simulink model "OMSv1_4"  (Simulink 7.0)
settings: Solver=ode4  SolverMode=SingleTasking  StartTime=0.0  StopTime=4  FixedStep=0.001  MaxStep=0.001  RelTol=1e-3  AbsTol=1e-3
PreLoadFcn:
  | setmdlp
values from neighbouring files (symbols this model uses):
  mdlparamlist = loadin.old    [setmdlp.m]
undefined symbols (not defined in the file or in its folder): alexlaw, bs_onoff, bs_scale, bsfsacrit, bsfsvcrit, cnsgain, current, fs_onoff, fs_scale, fsdelaycalc, ltdrk, phasicgain, pmcgain, pmctau2, pmctau3, saccsw, sigbuilder_block, spgain, tonicgain, tvrD, tvrN
(part 9 of 10)

== system OMSv1_4/OMS v1.4  12/31/07/IM CN-LMLN/Sampled Target Reconstruction/prolong/trailing edge detect/Sign ==
  in_1 : Inport  OutDataType=sfix(16)  OutScaling=2^0
  Constant : Constant  Value=0  OutDataType=sfix(16)  OutScaling=2^0
  Relational Operator : RelationalOperator  Operator=>  InputSameDT=on
  Relational Operator1 : RelationalOperator  Operator=<  InputSameDT=on
  Sum : Sum  Inputs=+-  OutDataType=sfix(16)  OutScaling=2^0  SaturateOnIntegerOverflow=on  InputSameDT=on
  out_1 : Outport  OutDataType=sfix(16)  OutScaling=2^0  InitialOutput=0
  wires:
  in_1/1 -> Relational Operator/1, Relational Operator1/1
  Constant/1 -> Relational Operator1/2, Relational Operator/2
  Relational Operator1/1 -> Sum/2
  Relational Operator/1 -> Sum/1
  Sum/1 -> out_1/1

== system OMSv1_4/OMS v1.4  12/31/07/IM CN-LMLN/Sampled Target Reconstruction/prolong1/SampHold?2/Sign ==
  in_1 : Inport  OutDataType=sfix(16)  OutScaling=2^0
  Constant : Constant  Value=0  OutDataType=sfix(16)  OutScaling=2^0
  Relational Operator : RelationalOperator  Operator=>  InputSameDT=on
  Relational Operator1 : RelationalOperator  Operator=<  InputSameDT=on
  Sum : Sum  Inputs=+-  OutDataType=sfix(16)  OutScaling=2^0  SaturateOnIntegerOverflow=on  InputSameDT=on
  out_1 : Outport  OutDataType=sfix(16)  OutScaling=2^0  InitialOutput=0
  wires:
  Sum/1 -> out_1/1
  Relational Operator/1 -> Sum/1
  Relational Operator1/1 -> Sum/2
  Constant/1 -> Relational Operator/2, Relational Operator1/2
  in_1/1 -> Relational Operator1/1, Relational Operator/1

== system OMSv1_4/OMS v1.4  12/31/07/IM CN-LMLN/Sampled Target Reconstruction/prolong1/leading edge detect/Sign ==
  in_1 : Inport  OutDataType=sfix(16)  OutScaling=2^0
  Constant : Constant  Value=0  OutDataType=sfix(16)  OutScaling=2^0
  Relational Operator : RelationalOperator  Operator=>  InputSameDT=on
  Relational Operator1 : RelationalOperator  Operator=<  InputSameDT=on
  Sum : Sum  Inputs=+-  OutDataType=sfix(16)  OutScaling=2^0  SaturateOnIntegerOverflow=on  InputSameDT=on
  out_1 : Outport  OutDataType=sfix(16)  OutScaling=2^0  InitialOutput=0
  wires:
  in_1/1 -> Relational Operator/1, Relational Operator1/1
  Constant/1 -> Relational Operator1/2, Relational Operator/2
  Relational Operator1/1 -> Sum/2
  Relational Operator/1 -> Sum/1
  Sum/1 -> out_1/1

== system OMSv1_4/OMS v1.4  12/31/07/IM CN-LMLN/Sampled Target Reconstruction/prolong1/trailing edge detect/Sign ==
  in_1 : Inport  OutDataType=sfix(16)  OutScaling=2^0
  Constant : Constant  Value=0  OutDataType=sfix(16)  OutScaling=2^0
  Relational Operator : RelationalOperator  Operator=>  InputSameDT=on
  Relational Operator1 : RelationalOperator  Operator=<  InputSameDT=on
  Sum : Sum  Inputs=+-  OutDataType=sfix(16)  OutScaling=2^0  SaturateOnIntegerOverflow=on  InputSameDT=on
  out_1 : Outport  OutDataType=sfix(16)  OutScaling=2^0  InitialOutput=0
  wires:
  Sum/1 -> out_1/1
  Relational Operator/1 -> Sum/1
  Relational Operator1/1 -> Sum/2
  Constant/1 -> Relational Operator/2, Relational Operator1/2
  in_1/1 -> Relational Operator1/1, Relational Operator/1

== system OMSv1_4/OMS v1.4  12/31/07/IM CN-LMLN/Sampled Target Reconstruction/prolong2/SampHold?2/Sign ==
  in_1 : Inport  OutDataType=sfix(16)  OutScaling=2^0
  Constant : Constant  Value=0  OutDataType=sfix(16)  OutScaling=2^0
  Relational Operator : RelationalOperator  Operator=>  InputSameDT=on
  Relational Operator1 : RelationalOperator  Operator=<  InputSameDT=on
  Sum : Sum  Inputs=+-  OutDataType=sfix(16)  OutScaling=2^0  SaturateOnIntegerOverflow=on  InputSameDT=on
  out_1 : Outport  OutDataType=sfix(16)  OutScaling=2^0  InitialOutput=0
  wires:
  in_1/1 -> Relational Operator/1, Relational Operator1/1
  Constant/1 -> Relational Operator1/2, Relational Operator/2
  Relational Operator1/1 -> Sum/2
  Relational Operator/1 -> Sum/1
  Sum/1 -> out_1/1

== system OMSv1_4/OMS v1.4  12/31/07/IM CN-LMLN/Sampled Target Reconstruction/prolong2/leading edge detect/Sign ==
  in_1 : Inport  OutDataType=sfix(16)  OutScaling=2^0
  Constant : Constant  Value=0  OutDataType=sfix(16)  OutScaling=2^0
  Relational Operator : RelationalOperator  Operator=>  InputSameDT=on
  Relational Operator1 : RelationalOperator  Operator=<  InputSameDT=on
  Sum : Sum  Inputs=+-  OutDataType=sfix(16)  OutScaling=2^0  SaturateOnIntegerOverflow=on  InputSameDT=on
  out_1 : Outport  OutDataType=sfix(16)  OutScaling=2^0  InitialOutput=0
  wires:
  Sum/1 -> out_1/1
  Relational Operator/1 -> Sum/1
  Relational Operator1/1 -> Sum/2
  Constant/1 -> Relational Operator/2, Relational Operator1/2
  in_1/1 -> Relational Operator1/1, Relational Operator/1

== system OMSv1_4/OMS v1.4  12/31/07/IM CN-LMLN/Sampled Target Reconstruction/prolong2/trailing edge detect/Sign ==
  in_1 : Inport  OutDataType=sfix(16)  OutScaling=2^0
  Constant : Constant  Value=0  OutDataType=sfix(16)  OutScaling=2^0
  Relational Operator : RelationalOperator  Operator=>  InputSameDT=on
  Relational Operator1 : RelationalOperator  Operator=<  InputSameDT=on
  Sum : Sum  Inputs=+-  OutDataType=sfix(16)  OutScaling=2^0  SaturateOnIntegerOverflow=on  InputSameDT=on
  out_1 : Outport  OutDataType=sfix(16)  OutScaling=2^0  InitialOutput=0
  wires:
  in_1/1 -> Relational Operator/1, Relational Operator1/1
  Constant/1 -> Relational Operator1/2, Relational Operator/2
  Relational Operator1/1 -> Sum/2
  Relational Operator/1 -> Sum/1
  Sum/1 -> out_1/1

== system OMSv1_4/OMS v1.4  12/31/07/PG w rNI2/PW funct/Input Switch/lead/trail edge det/Sign ==
  in_1 : Inport  OutDataType=sfix(16)  OutScaling=2^0
  Constant : Constant  Value=0  OutDataType=sfix(16)  OutScaling=2^0
  Relational Operator : RelationalOperator  Operator=>  InputSameDT=on
  Relational Operator1 : RelationalOperator  Operator=<  InputSameDT=on
  Sum : Sum  Inputs=+-  OutDataType=sfix(16)  OutScaling=2^0  SaturateOnIntegerOverflow=on  InputSameDT=on
  out_1 : Outport  OutDataType=sfix(16)  OutScaling=2^0  InitialOutput=0
  wires:
  in_1/1 -> Relational Operator/1, Relational Operator1/1
  Constant/1 -> Relational Operator1/2, Relational Operator/2
  Relational Operator1/1 -> Sum/2
  Relational Operator/1 -> Sum/1
  Sum/1 -> out_1/1

== system OMSv1_4/OMS v1.4  12/31/07/PG w rNI2/RefLatch (Default = 50ms)/trailing edge/trailing edge det/Sign ==
  in_1 : Inport  OutDataType=sfix(16)  OutScaling=2^0
  Constant : Constant  Value=0  OutDataType=sfix(16)  OutScaling=2^0
  Relational Operator : RelationalOperator  Operator=>  InputSameDT=on
  Relational Operator1 : RelationalOperator  Operator=<  InputSameDT=on
  Sum : Sum  Inputs=+-  OutDataType=sfix(16)  OutScaling=2^0  SaturateOnIntegerOverflow=on  InputSameDT=on
  out_1 : Outport  OutDataType=sfix(16)  OutScaling=2^0  InitialOutput=0
  wires:
  in_1/1 -> Relational Operator/1, Relational Operator1/1
  Constant/1 -> Relational Operator1/2, Relational Operator/2
  Relational Operator1/1 -> Sum/2
  Relational Operator/1 -> Sum/1
  Sum/1 -> out_1/1

== system OMSv1_4/OMS v1.4  12/31/07/PG w rNI2/RefLatch (Default = 50ms)/trailing edge/trailing edge det1/Sign ==
  in_1 : Inport  OutDataType=sfix(16)  OutScaling=2^0
  Constant : Constant  Value=0  OutDataType=sfix(16)  OutScaling=2^0
  Relational Operator : RelationalOperator  Operator=>  InputSameDT=on
  Relational Operator1 : RelationalOperator  Operator=<  InputSameDT=on
  Sum : Sum  Inputs=+-  OutDataType=sfix(16)  OutScaling=2^0  SaturateOnIntegerOverflow=on  InputSameDT=on
  out_1 : Outport  OutDataType=sfix(16)  OutScaling=2^0  InitialOutput=0
  wires:
  Sum/1 -> out_1/1
  Relational Operator/1 -> Sum/1
  Relational Operator1/1 -> Sum/2
  Constant/1 -> Relational Operator1/2, Relational Operator/2
  in_1/1 -> Relational Operator/1, Relational Operator1/1

== system OMSv1_4/OMS v1.4  12/31/07/IM CN-LMLN/BS/FS Logic/BS Enable1/BS Timing/event timer2/Latch1 ==
  in_1 : Inport  OutDataType=sfix(16)  OutScaling=2^0
  in_2 : Inport  Port=2  OutDataType=sfix(16)  OutScaling=2^0
  Demux : Demux  Outputs=2
  Logic : CombinatorialLogic  TruthTable=[0 1;0 1;1 0;0 1;1 0;0 1;1 0;1 0]
  Memory : Memory  Orientation=left  X0=ini
  Mux : Mux  Inputs=3
  out_1 : Outport  OutDataType=sfix(16)  OutScaling=2^0  InitialOutput=0
  out_2 : Outport  Port=2  OutDataType=sfix(16)  OutScaling=2^0  InitialOutput=0
  wires:
  in_2/1 -> Mux/3
  in_1/1 -> Mux/2
  Memory/1 -> Mux/1
  Demux/1 -> Memory/1, out_1/1
  Mux/1 -> Logic/1
  Logic/1 -> Demux/1
  Demux/2 -> out_2/1

== system OMSv1_4/OMS v1.4  12/31/07/IM CN-LMLN/BS/FS Logic/BS Enable1/BS Timing/event timer2/SampHold?1 ==
  note: When "S/H?" is LOW, then "Input" is switched directly to the
      | output ("sample").  When "S/H?" is HIGH, the current output is
      | maintained ("hold").
  Input : Inport  OutDataType=sfix(16)  OutScaling=2^0
  S/H? : Inport  Port=2  OutDataType=sfix(16)  OutScaling=2^0
  Memory : Memory  Orientation=left
  Sign : Subsystem
      mask Type: Sign
      mask Description: y = sign(x)
      mask Help: Sign Function:\n\t\t\ty = 1 if x > 0\n\t\t\ty = 0 if x = 0\n\t\t\ty = -1 if x < 0
      mask Display: plot(-50,-50,50,50,[-50,50],[0,0],[0,0],[-50,50],[-40,0],[-30,-30],[0,40],[30,30])
  Switch2 : Switch  Threshold=0.5  SaturateOnIntegerOverflow=on  InputSameDT=on
  output : Outport  OutDataType=sfix(16)  OutScaling=2^0  InitialOutput=0
  wires:
  Switch2/1 -> Memory/1, output/1
  Sign/1(out_1) -> Switch2/2
  S/H?/1 -> Sign/1(in_1)
  Memory/1 -> Switch2/1
  Input/1 -> Switch2/3

== system OMSv1_4/OMS v1.4  12/31/07/IM CN-LMLN/BS/FS Logic/BS Enable1/BS Timing/event timer2/leading edge detect ==
  note: It is also possible to remove the SIGNUM function
      | and the '==', and replace them with a simple
      | switch with a threshold of (say) 150 or so.
  note: leading edge detection
  in_1 : Inport  OutDataType=sfix(16)  OutScaling=2^0
  Abs : Abs  SaturateOnIntegerOverflow=on
  Derivative : Derivative
  Relational Operator : RelationalOperator  Operator===  InputSameDT=on
  Sign : Subsystem
      mask Type: Sign
      mask Description: y = sign(x)
      mask Help: Sign Function:\n\t\t\ty = 1 if x > 0\n\t\t\ty = 0 if x = 0\n\t\t\ty = -1 if x < 0
      mask Display: plot(-50,-50,50,50,[-50,50],[0,0],[0,0],[-50,50],[-40,0],[-30,-30],[0,40],[30,30])
  Threshold 1 : Constant  OutDataType=sfix(16)  OutScaling=2^0
  out_1 : Outport  OutDataType=sfix(16)  OutScaling=2^0  InitialOutput=0
  wires:
  Abs/1 -> Derivative/1
  Derivative/1 -> Sign/1(in_1)
  Sign/1(out_1) -> Relational Operator/1
  Threshold 1/1 -> Relational Operator/2
  Relational Operator/1 -> out_1/1
  in_1/1 -> Abs/1

== system OMSv1_4/OMS v1.4  12/31/07/IM CN-LMLN/BS/FS Logic/BS Enable1/BS Timing/event timer2/trailing edge detect ==
  note: trailing edge detection
  note: It is also possible to remove the SIGNUM function
      | and the '==', and replace them with a simple
      | switch with a threshold of (say) 150 or so.
  in_1 : Inport  OutDataType=sfix(16)  OutScaling=2^0
  Abs : Abs  SaturateOnIntegerOverflow=on
  Derivative : Derivative
  Relational Operator : RelationalOperator  Operator===  InputSameDT=on
  Sign : Subsystem
      mask Type: Sign
      mask Description: y = sign(x)
      mask Help: Sign Function:\n\t\t\ty = 1 if x > 0\n\t\t\ty = 0 if x = 0\n\t\t\ty = -1 if x < 0
      mask Display: plot(-50,-50,50,50,[-50,50],[0,0],[0,0],[-50,50],[-40,0],[-30,-30],[0,40],[30,30])
  Threshold 1 : Constant  Value=-1  OutDataType=sfix(16)  OutScaling=2^0
  out_1 : Outport  OutDataType=sfix(16)  OutScaling=2^0  InitialOutput=0
  wires:
  in_1/1 -> Abs/1
  Relational Operator/1 -> out_1/1
  Threshold 1/1 -> Relational Operator/2
  Sign/1(out_1) -> Relational Operator/1
  Derivative/1 -> Sign/1(in_1)
  Abs/1 -> Derivative/1

== system OMSv1_4/OMS v1.4  12/31/07/IM CN-LMLN/BS/FS Logic/BS Enable1/BS Timing/leading edge detect/Sign ==
  in_1 : Inport  OutDataType=sfix(16)  OutScaling=2^0
  Constant : Constant  Value=0  OutDataType=sfix(16)  OutScaling=2^0
  Relational Operator : RelationalOperator  Operator=>  InputSameDT=on
  Relational Operator1 : RelationalOperator  Operator=<  InputSameDT=on
  Sum : Sum  Inputs=+-  OutDataType=sfix(16)  OutScaling=2^0  SaturateOnIntegerOverflow=on  InputSameDT=on
  out_1 : Outport  OutDataType=sfix(16)  OutScaling=2^0  InitialOutput=0
  wires:
  Sum/1 -> out_1/1
  Relational Operator/1 -> Sum/1
  Relational Operator1/1 -> Sum/2
  Constant/1 -> Relational Operator/2, Relational Operator1/2
  in_1/1 -> Relational Operator1/1, Relational Operator/1

== system OMSv1_4/OMS v1.4  12/31/07/IM CN-LMLN/BS/FS Logic/FS Enable/FS Timing/event timer2/Latch1 ==
  in_1 : Inport  OutDataType=sfix(16)  OutScaling=2^0
  in_2 : Inport  Port=2  OutDataType=sfix(16)  OutScaling=2^0
  Demux : Demux  Outputs=2
  Logic : CombinatorialLogic  TruthTable=[0 1;0 1;1 0;0 1;1 0;0 1;1 0;1 0]
  Memory : Memory  Orientation=left  X0=ini
  Mux : Mux  Inputs=3
  out_1 : Outport  OutDataType=sfix(16)  OutScaling=2^0  InitialOutput=0
  out_2 : Outport  Port=2  OutDataType=sfix(16)  OutScaling=2^0  InitialOutput=0
  wires:
  Demux/2 -> out_2/1
  Logic/1 -> Demux/1
  Mux/1 -> Logic/1
  Demux/1 -> out_1/1, Memory/1
  Memory/1 -> Mux/1
  in_1/1 -> Mux/2
  in_2/1 -> Mux/3

== system OMSv1_4/OMS v1.4  12/31/07/IM CN-LMLN/BS/FS Logic/FS Enable/FS Timing/event timer2/SampHold?1 ==
  note: When "S/H?" is LOW, then "Input" is switched directly to the
      | output ("sample").  When "S/H?" is HIGH, the current output is
      | maintained ("hold").
  Input : Inport  OutDataType=sfix(16)  OutScaling=2^0
  S/H? : Inport  Port=2  OutDataType=sfix(16)  OutScaling=2^0
  Memory : Memory  Orientation=left
  Sign : Subsystem
      mask Type: Sign
      mask Description: y = sign(x)
      mask Help: Sign Function:\n\t\t\ty = 1 if x > 0\n\t\t\ty = 0 if x = 0\n\t\t\ty = -1 if x < 0
      mask Display: plot(-50,-50,50,50,[-50,50],[0,0],[0,0],[-50,50],[-40,0],[-30,-30],[0,40],[30,30])
  Switch2 : Switch  Threshold=0.5  SaturateOnIntegerOverflow=on  InputSameDT=on
  output : Outport  OutDataType=sfix(16)  OutScaling=2^0  InitialOutput=0
  wires:
  Input/1 -> Switch2/3
  Memory/1 -> Switch2/1
  S/H?/1 -> Sign/1(in_1)
  Sign/1(out_1) -> Switch2/2
  Switch2/1 -> output/1, Memory/1

== system OMSv1_4/OMS v1.4  12/31/07/IM CN-LMLN/BS/FS Logic/FS Enable/FS Timing/event timer2/leading edge detect ==
  note: leading edge detection
  note: It is also possible to remove the SIGNUM function
      | and the '==', and replace them with a simple
      | switch with a threshold of (say) 150 or so.
  in_1 : Inport  OutDataType=sfix(16)  OutScaling=2^0
  Abs : Abs  SaturateOnIntegerOverflow=on
  Derivative : Derivative
  Relational Operator : RelationalOperator  Operator===  InputSameDT=on
  Sign : Subsystem
      mask Type: Sign
      mask Description: y = sign(x)
      mask Help: Sign Function:\n\t\t\ty = 1 if x > 0\n\t\t\ty = 0 if x = 0\n\t\t\ty = -1 if x < 0
      mask Display: plot(-50,-50,50,50,[-50,50],[0,0],[0,0],[-50,50],[-40,0],[-30,-30],[0,40],[30,30])
  Threshold 1 : Constant  OutDataType=sfix(16)  OutScaling=2^0
  out_1 : Outport  OutDataType=sfix(16)  OutScaling=2^0  InitialOutput=0
  wires:
  in_1/1 -> Abs/1
  Relational Operator/1 -> out_1/1
  Threshold 1/1 -> Relational Operator/2
  Sign/1(out_1) -> Relational Operator/1
  Derivative/1 -> Sign/1(in_1)
  Abs/1 -> Derivative/1

== system OMSv1_4/OMS v1.4  12/31/07/IM CN-LMLN/BS/FS Logic/FS Enable/FS Timing/event timer2/trailing edge detect ==
  note: It is also possible to remove the SIGNUM function
      | and the '==', and replace them with a simple
      | switch with a threshold of (say) 150 or so.
  note: trailing edge detection
  in_1 : Inport  OutDataType=sfix(16)  OutScaling=2^0
  Abs : Abs  SaturateOnIntegerOverflow=on
  Derivative : Derivative
  Relational Operator : RelationalOperator  Operator===  InputSameDT=on
  Sign : Subsystem
      mask Type: Sign
      mask Description: y = sign(x)
      mask Help: Sign Function:\n\t\t\ty = 1 if x > 0\n\t\t\ty = 0 if x = 0\n\t\t\ty = -1 if x < 0
      mask Display: plot(-50,-50,50,50,[-50,50],[0,0],[0,0],[-50,50],[-40,0],[-30,-30],[0,40],[30,30])
  Threshold 1 : Constant  Value=-1  OutDataType=sfix(16)  OutScaling=2^0
  out_1 : Outport  OutDataType=sfix(16)  OutScaling=2^0  InitialOutput=0
  wires:
  Abs/1 -> Derivative/1
  Derivative/1 -> Sign/1(in_1)
  Sign/1(out_1) -> Relational Operator/1
  Threshold 1/1 -> Relational Operator/2
  Relational Operator/1 -> out_1/1
  in_1/1 -> Abs/1

== system OMSv1_4/OMS v1.4  12/31/07/IM CN-LMLN/BS/FS Logic/FS Enable/FS Timing/leading edge detect/Sign ==
  in_1 : Inport  OutDataType=sfix(16)  OutScaling=2^0
  Constant : Constant  Value=0  OutDataType=sfix(16)  OutScaling=2^0
  Relational Operator : RelationalOperator  Operator=>  InputSameDT=on
  Relational Operator1 : RelationalOperator  Operator=<  InputSameDT=on
  Sum : Sum  Inputs=+-  OutDataType=sfix(16)  OutScaling=2^0  SaturateOnIntegerOverflow=on  InputSameDT=on
  out_1 : Outport  OutDataType=sfix(16)  OutScaling=2^0  InitialOutput=0
  wires:
  in_1/1 -> Relational Operator/1, Relational Operator1/1
  Constant/1 -> Relational Operator1/2, Relational Operator/2
  Relational Operator1/1 -> Sum/2
  Relational Operator/1 -> Sum/1
  Sum/1 -> out_1/1

== system OMSv1_4/OMS v1.4  12/31/07/IM CN-LMLN/BS/FS Logic/FS Enable/prolong/SampHold?2/Sign ==
  in_1 : Inport  OutDataType=sfix(16)  OutScaling=2^0
  Constant : Constant  Value=0  OutDataType=sfix(16)  OutScaling=2^0
  Relational Operator : RelationalOperator  Operator=>  InputSameDT=on
  Relational Operator1 : RelationalOperator  Operator=<  InputSameDT=on
  Sum : Sum  Inputs=+-  OutDataType=sfix(16)  OutScaling=2^0  SaturateOnIntegerOverflow=on  InputSameDT=on
  out_1 : Outport  OutDataType=sfix(16)  OutScaling=2^0  InitialOutput=0
  wires:
  in_1/1 -> Relational Operator/1, Relational Operator1/1
  Constant/1 -> Relational Operator1/2, Relational Operator/2
  Relational Operator1/1 -> Sum/2
  Relational Operator/1 -> Sum/1
  Sum/1 -> out_1/1

== system OMSv1_4/OMS v1.4  12/31/07/IM CN-LMLN/BS/FS Logic/FS Enable/prolong/leading edge detect/Sign ==
  in_1 : Inport  OutDataType=sfix(16)  OutScaling=2^0
  Constant : Constant  Value=0  OutDataType=sfix(16)  OutScaling=2^0
  Relational Operator : RelationalOperator  Operator=>  InputSameDT=on
  Relational Operator1 : RelationalOperator  Operator=<  InputSameDT=on
  Sum : Sum  Inputs=+-  OutDataType=sfix(16)  OutScaling=2^0  SaturateOnIntegerOverflow=on  InputSameDT=on
  out_1 : Outport  OutDataType=sfix(16)  OutScaling=2^0  InitialOutput=0
  wires:
  Sum/1 -> out_1/1
  Relational Operator/1 -> Sum/1
  Relational Operator1/1 -> Sum/2
  Constant/1 -> Relational Operator/2, Relational Operator1/2
  in_1/1 -> Relational Operator1/1, Relational Operator/1

== system OMSv1_4/OMS v1.4  12/31/07/IM CN-LMLN/BS/FS Logic/FS Enable/prolong/trailing edge detect/Sign ==
  in_1 : Inport  OutDataType=sfix(16)  OutScaling=2^0
  Constant : Constant  Value=0  OutDataType=sfix(16)  OutScaling=2^0
  Relational Operator : RelationalOperator  Operator=>  InputSameDT=on
  Relational Operator1 : RelationalOperator  Operator=<  InputSameDT=on
  Sum : Sum  Inputs=+-  OutDataType=sfix(16)  OutScaling=2^0  SaturateOnIntegerOverflow=on  InputSameDT=on
  out_1 : Outport  OutDataType=sfix(16)  OutScaling=2^0  InitialOutput=0
  wires:
  in_1/1 -> Relational Operator/1, Relational Operator1/1
  Constant/1 -> Relational Operator1/2, Relational Operator/2
  Relational Operator1/1 -> Sum/2
  Relational Operator/1 -> Sum/1
  Sum/1 -> out_1/1

== system OMSv1_4/OMS v1.4  12/31/07/IM CN-LMLN/BS/FS Logic/TCHNG Override/event timer2/SampHold?1/Sign ==
  in_1 : Inport  OutDataType=sfix(16)  OutScaling=2^0
  Constant : Constant  Value=0  OutDataType=sfix(16)  OutScaling=2^0
  Relational Operator : RelationalOperator  Operator=>  InputSameDT=on
  Relational Operator1 : RelationalOperator  Operator=<  InputSameDT=on
  Sum : Sum  Inputs=+-  OutDataType=sfix(16)  OutScaling=2^0  SaturateOnIntegerOverflow=on  InputSameDT=on
  out_1 : Outport  OutDataType=sfix(16)  OutScaling=2^0  InitialOutput=0
  wires:
  in_1/1 -> Relational Operator1/1, Relational Operator/1
  Constant/1 -> Relational Operator/2, Relational Operator1/2
  Relational Operator1/1 -> Sum/2
  Relational Operator/1 -> Sum/1
  Sum/1 -> out_1/1

== system OMSv1_4/OMS v1.4  12/31/07/IM CN-LMLN/BS/FS Logic/TCHNG Override/event timer2/leading edge detect/Sign ==
  in_1 : Inport  OutDataType=sfix(16)  OutScaling=2^0
  Constant : Constant  Value=0  OutDataType=sfix(16)  OutScaling=2^0
  Relational Operator : RelationalOperator  Operator=>  InputSameDT=on
  Relational Operator1 : RelationalOperator  Operator=<  InputSameDT=on
  Sum : Sum  Inputs=+-  OutDataType=sfix(16)  OutScaling=2^0  SaturateOnIntegerOverflow=on  InputSameDT=on
  out_1 : Outport  OutDataType=sfix(16)  OutScaling=2^0  InitialOutput=0
  wires:
  in_1/1 -> Relational Operator1/1, Relational Operator/1
  Constant/1 -> Relational Operator/2, Relational Operator1/2
  Relational Operator1/1 -> Sum/2
  Relational Operator/1 -> Sum/1
  Sum/1 -> out_1/1

== system OMSv1_4/OMS v1.4  12/31/07/IM CN-LMLN/BS/FS Logic/TCHNG Override/event timer2/trailing edge detect/Sign ==
  in_1 : Inport  OutDataType=sfix(16)  OutScaling=2^0
  Constant : Constant  Value=0  OutDataType=sfix(16)  OutScaling=2^0
  Relational Operator : RelationalOperator  Operator=>  InputSameDT=on
  Relational Operator1 : RelationalOperator  Operator=<  InputSameDT=on
  Sum : Sum  Inputs=+-  OutDataType=sfix(16)  OutScaling=2^0  SaturateOnIntegerOverflow=on  InputSameDT=on
  out_1 : Outport  OutDataType=sfix(16)  OutScaling=2^0  InitialOutput=0
  wires:
  Sum/1 -> out_1/1
  Relational Operator/1 -> Sum/1
  Relational Operator1/1 -> Sum/2
  Constant/1 -> Relational Operator/2, Relational Operator1/2
  in_1/1 -> Relational Operator1/1, Relational Operator/1

== system OMSv1_4/OMS v1.4  12/31/07/IM CN-LMLN/Saccade Enable/Enable Control/2 ms/SampHold?2/Sign ==
  in_1 : Inport  OutDataType=sfix(16)  OutScaling=2^0
  Constant : Constant  Value=0  OutDataType=sfix(16)  OutScaling=2^0
  Relational Operator : RelationalOperator  Operator=>  InputSameDT=on
  Relational Operator1 : RelationalOperator  Operator=<  InputSameDT=on
  Sum : Sum  Inputs=+-  OutDataType=sfix(16)  OutScaling=2^0  SaturateOnIntegerOverflow=on  InputSameDT=on
  out_1 : Outport  OutDataType=sfix(16)  OutScaling=2^0  InitialOutput=0
  wires:
  Sum/1 -> out_1/1
  Relational Operator/1 -> Sum/1
  Relational Operator1/1 -> Sum/2
  Constant/1 -> Relational Operator/2, Relational Operator1/2
  in_1/1 -> Relational Operator1/1, Relational Operator/1

== system OMSv1_4/OMS v1.4  12/31/07/IM CN-LMLN/Saccade Enable/Enable Control/2 ms/leading edge detect/Sign ==
  in_1 : Inport  OutDataType=sfix(16)  OutScaling=2^0
  Constant : Constant  Value=0  OutDataType=sfix(16)  OutScaling=2^0
  Relational Operator : RelationalOperator  Operator=>  InputSameDT=on
  Relational Operator1 : RelationalOperator  Operator=<  InputSameDT=on
  Sum : Sum  Inputs=+-  OutDataType=sfix(16)  OutScaling=2^0  SaturateOnIntegerOverflow=on  InputSameDT=on
  out_1 : Outport  OutDataType=sfix(16)  OutScaling=2^0  InitialOutput=0
  wires:
  in_1/1 -> Relational Operator/1, Relational Operator1/1
  Constant/1 -> Relational Operator1/2, Relational Operator/2
  Relational Operator1/1 -> Sum/2
  Relational Operator/1 -> Sum/1
  Sum/1 -> out_1/1

== system OMSv1_4/OMS v1.4  12/31/07/IM CN-LMLN/Saccade Enable/Enable Control/2 ms/trailing edge detect/Sign ==
  in_1 : Inport  OutDataType=sfix(16)  OutScaling=2^0
  Constant : Constant  Value=0  OutDataType=sfix(16)  OutScaling=2^0
  Relational Operator : RelationalOperator  Operator=>  InputSameDT=on
  Relational Operator1 : RelationalOperator  Operator=<  InputSameDT=on
  Sum : Sum  Inputs=+-  OutDataType=sfix(16)  OutScaling=2^0  SaturateOnIntegerOverflow=on  InputSameDT=on
  out_1 : Outport  OutDataType=sfix(16)  OutScaling=2^0  InitialOutput=0
  wires:
  Sum/1 -> out_1/1
  Relational Operator/1 -> Sum/1
  Relational Operator1/1 -> Sum/2
  Constant/1 -> Relational Operator/2, Relational Operator1/2
  in_1/1 -> Relational Operator1/1, Relational Operator/1

== system OMSv1_4/OMS v1.4  12/31/07/IM CN-LMLN/Saccade Enable/Enable Control/50 ms/SampHold?2/Sign ==
  in_1 : Inport  OutDataType=sfix(16)  OutScaling=2^0
  Constant : Constant  Value=0  OutDataType=sfix(16)  OutScaling=2^0
  Relational Operator : RelationalOperator  Operator=>  InputSameDT=on
  Relational Operator1 : RelationalOperator  Operator=<  InputSameDT=on
  Sum : Sum  Inputs=+-  OutDataType=sfix(16)  OutScaling=2^0  SaturateOnIntegerOverflow=on  InputSameDT=on
  out_1 : Outport  OutDataType=sfix(16)  OutScaling=2^0  InitialOutput=0
  wires:
  in_1/1 -> Relational Operator/1, Relational Operator1/1
  Constant/1 -> Relational Operator1/2, Relational Operator/2
  Relational Operator1/1 -> Sum/2
  Relational Operator/1 -> Sum/1
  Sum/1 -> out_1/1

== system OMSv1_4/OMS v1.4  12/31/07/IM CN-LMLN/Saccade Enable/Enable Control/50 ms/leading edge detect/Sign ==
  in_1 : Inport  OutDataType=sfix(16)  OutScaling=2^0
  Constant : Constant  Value=0  OutDataType=sfix(16)  OutScaling=2^0
  Relational Operator : RelationalOperator  Operator=>  InputSameDT=on
  Relational Operator1 : RelationalOperator  Operator=<  InputSameDT=on
  Sum : Sum  Inputs=+-  OutDataType=sfix(16)  OutScaling=2^0  SaturateOnIntegerOverflow=on  InputSameDT=on
  out_1 : Outport  OutDataType=sfix(16)  OutScaling=2^0  InitialOutput=0
  wires:
  Sum/1 -> out_1/1
  Relational Operator/1 -> Sum/1
  Relational Operator1/1 -> Sum/2
  Constant/1 -> Relational Operator/2, Relational Operator1/2
  in_1/1 -> Relational Operator1/1, Relational Operator/1

== system OMSv1_4/OMS v1.4  12/31/07/IM CN-LMLN/Saccade Enable/Enable Control/50 ms/trailing edge detect/Sign ==
  in_1 : Inport  OutDataType=sfix(16)  OutScaling=2^0
  Constant : Constant  Value=0  OutDataType=sfix(16)  OutScaling=2^0
  Relational Operator : RelationalOperator  Operator=>  InputSameDT=on
  Relational Operator1 : RelationalOperator  Operator=<  InputSameDT=on
  Sum : Sum  Inputs=+-  OutDataType=sfix(16)  OutScaling=2^0  SaturateOnIntegerOverflow=on  InputSameDT=on
  out_1 : Outport  OutDataType=sfix(16)  OutScaling=2^0  InitialOutput=0
  wires:
  in_1/1 -> Relational Operator/1, Relational Operator1/1
  Constant/1 -> Relational Operator1/2, Relational Operator/2
  Relational Operator1/1 -> Sum/2
  Relational Operator/1 -> Sum/1
  Sum/1 -> out_1/1

== system OMSv1_4/OMS v1.4  12/31/07/IM CN-LMLN/Saccade Enable/Enable Control/ECPY Timing/leading edge detect/Sign ==
  in_1 : Inport  OutDataType=sfix(16)  OutScaling=2^0
  Constant : Constant  Value=0  OutDataType=sfix(16)  OutScaling=2^0
  Relational Operator : RelationalOperator  Operator=>  InputSameDT=on
  Relational Operator1 : RelationalOperator  Operator=<  InputSameDT=on
  Sum : Sum  Inputs=+-  OutDataType=sfix(16)  OutScaling=2^0  SaturateOnIntegerOverflow=on  InputSameDT=on
  out_1 : Outport  OutDataType=sfix(16)  OutScaling=2^0  InitialOutput=0
  wires:
  in_1/1 -> Relational Operator1/1, Relational Operator/1
  Constant/1 -> Relational Operator/2, Relational Operator1/2
  Relational Operator1/1 -> Sum/2
  Relational Operator/1 -> Sum/1
  Sum/1 -> out_1/1

== system OMSv1_4/OMS v1.4  12/31/07/IM CN-LMLN/Saccade Enable/Enable Control/ECPY Timing/leading edge detect1/Sign ==
  in_1 : Inport  OutDataType=sfix(16)  OutScaling=2^0
  Constant : Constant  Value=0  OutDataType=sfix(16)  OutScaling=2^0
  Relational Operator : RelationalOperator  Operator=>  InputSameDT=on
  Relational Operator1 : RelationalOperator  Operator=<  InputSameDT=on
  Sum : Sum  Inputs=+-  OutDataType=sfix(16)  OutScaling=2^0  SaturateOnIntegerOverflow=on  InputSameDT=on
  out_1 : Outport  OutDataType=sfix(16)  OutScaling=2^0  InitialOutput=0
  wires:
  Sum/1 -> out_1/1
  Relational Operator/1 -> Sum/1
  Relational Operator1/1 -> Sum/2
  Constant/1 -> Relational Operator/2, Relational Operator1/2
  in_1/1 -> Relational Operator1/1, Relational Operator/1

== system OMSv1_4/OMS v1.4  12/31/07/IM CN-LMLN/Saccade Enable/Enable Control/ECPY Timing/trailing edge detect/Sign ==
  in_1 : Inport  OutDataType=sfix(16)  OutScaling=2^0
  Constant : Constant  Value=0  OutDataType=sfix(16)  OutScaling=2^0
  Relational Operator : RelationalOperator  Operator=>  InputSameDT=on
  Relational Operator1 : RelationalOperator  Operator=<  InputSameDT=on
  Sum : Sum  Inputs=+-  OutDataType=sfix(16)  OutScaling=2^0  SaturateOnIntegerOverflow=on  InputSameDT=on
  out_1 : Outport  OutDataType=sfix(16)  OutScaling=2^0  InitialOutput=0
  wires:
  Sum/1 -> out_1/1
  Relational Operator/1 -> Sum/1
  Relational Operator1/1 -> Sum/2
  Constant/1 -> Relational Operator/2, Relational Operator1/2
  in_1/1 -> Relational Operator1/1, Relational Operator/1

== system OMSv1_4/OMS v1.4  12/31/07/IM CN-LMLN/Saccade Enable/Enable Control/event timer1/SampHold?1/Sign ==
  in_1 : Inport  OutDataType=sfix(16)  OutScaling=2^0
  Constant : Constant  Value=0  OutDataType=sfix(16)  OutScaling=2^0
  Relational Operator : RelationalOperator  Operator=>  InputSameDT=on
  Relational Operator1 : RelationalOperator  Operator=<  InputSameDT=on
  Sum : Sum  Inputs=+-  OutDataType=sfix(16)  OutScaling=2^0  SaturateOnIntegerOverflow=on  InputSameDT=on
  out_1 : Outport  OutDataType=sfix(16)  OutScaling=2^0  InitialOutput=0
  wires:
  Sum/1 -> out_1/1
  Relational Operator/1 -> Sum/1
  Relational Operator1/1 -> Sum/2
  Constant/1 -> Relational Operator/2, Relational Operator1/2
  in_1/1 -> Relational Operator1/1, Relational Operator/1

== system OMSv1_4/OMS v1.4  12/31/07/IM CN-LMLN/Saccade Enable/Enable Control/event timer1/leading edge detect/Sign ==
  in_1 : Inport  OutDataType=sfix(16)  OutScaling=2^0
  Constant : Constant  Value=0  OutDataType=sfix(16)  OutScaling=2^0
  Relational Operator : RelationalOperator  Operator=>  InputSameDT=on
  Relational Operator1 : RelationalOperator  Operator=<  InputSameDT=on
  Sum : Sum  Inputs=+-  OutDataType=sfix(16)  OutScaling=2^0  SaturateOnIntegerOverflow=on  InputSameDT=on
  out_1 : Outport  OutDataType=sfix(16)  OutScaling=2^0  InitialOutput=0
  wires:
  Sum/1 -> out_1/1
  Relational Operator/1 -> Sum/1
  Relational Operator1/1 -> Sum/2
  Constant/1 -> Relational Operator/2, Relational Operator1/2
  in_1/1 -> Relational Operator1/1, Relational Operator/1

== system OMSv1_4/OMS v1.4  12/31/07/IM CN-LMLN/Saccade Enable/Enable Control/event timer1/trailing edge detect/Sign ==
  in_1 : Inport  OutDataType=sfix(16)  OutScaling=2^0
  Constant : Constant  Value=0  OutDataType=sfix(16)  OutScaling=2^0
  Relational Operator : RelationalOperator  Operator=>  InputSameDT=on
  Relational Operator1 : RelationalOperator  Operator=<  InputSameDT=on
  Sum : Sum  Inputs=+-  OutDataType=sfix(16)  OutScaling=2^0  SaturateOnIntegerOverflow=on  InputSameDT=on
  out_1 : Outport  OutDataType=sfix(16)  OutScaling=2^0  InitialOutput=0
  wires:
  in_1/1 -> Relational Operator1/1, Relational Operator/1
  Constant/1 -> Relational Operator/2, Relational Operator1/2
  Relational Operator1/1 -> Sum/2
  Relational Operator/1 -> Sum/1
  Sum/1 -> out_1/1

== system OMSv1_4/OMS v1.4  12/31/07/IM CN-LMLN/Saccade Enable/LN FPh Gen/event timer1/SampHold?1/Sign ==
  in_1 : Inport  OutDataType=sfix(16)  OutScaling=2^0
  Constant : Constant  Value=0  OutDataType=sfix(16)  OutScaling=2^0
  Relational Operator : RelationalOperator  Operator=>  InputSameDT=on
  Relational Operator1 : RelationalOperator  Operator=<  InputSameDT=on
  Sum : Sum  Inputs=+-  OutDataType=sfix(16)  OutScaling=2^0  SaturateOnIntegerOverflow=on  InputSameDT=on
  out_1 : Outport  OutDataType=sfix(16)  OutScaling=2^0  InitialOutput=0
  wires:
  Sum/1 -> out_1/1
  Relational Operator/1 -> Sum/1
  Relational Operator1/1 -> Sum/2
  Constant/1 -> Relational Operator/2, Relational Operator1/2
  in_1/1 -> Relational Operator1/1, Relational Operator/1

== system OMSv1_4/OMS v1.4  12/31/07/IM CN-LMLN/Saccade Enable/LN FPh Gen/event timer1/leading edge detect/Sign ==
  in_1 : Inport  OutDataType=sfix(16)  OutScaling=2^0
  Constant : Constant  Value=0  OutDataType=sfix(16)  OutScaling=2^0
  Relational Operator : RelationalOperator  Operator=>  InputSameDT=on
  Relational Operator1 : RelationalOperator  Operator=<  InputSameDT=on
  Sum : Sum  Inputs=+-  OutDataType=sfix(16)  OutScaling=2^0  SaturateOnIntegerOverflow=on  InputSameDT=on
  out_1 : Outport  OutDataType=sfix(16)  OutScaling=2^0  InitialOutput=0
  wires:
  Sum/1 -> out_1/1
  Relational Operator/1 -> Sum/1
  Relational Operator1/1 -> Sum/2
  Constant/1 -> Relational Operator/2, Relational Operator1/2
  in_1/1 -> Relational Operator1/1, Relational Operator/1

== system OMSv1_4/OMS v1.4  12/31/07/IM CN-LMLN/Saccade Enable/LN FPh Gen/event timer1/trailing edge detect/Sign ==
  in_1 : Inport  OutDataType=sfix(16)  OutScaling=2^0
  Constant : Constant  Value=0  OutDataType=sfix(16)  OutScaling=2^0
  Relational Operator : RelationalOperator  Operator=>  InputSameDT=on
  Relational Operator1 : RelationalOperator  Operator=<  InputSameDT=on
  Sum : Sum  Inputs=+-  OutDataType=sfix(16)  OutScaling=2^0  SaturateOnIntegerOverflow=on  InputSameDT=on
  out_1 : Outport  OutDataType=sfix(16)  OutScaling=2^0  InitialOutput=0
  wires:
  in_1/1 -> Relational Operator1/1, Relational Operator/1
  Constant/1 -> Relational Operator/2, Relational Operator1/2
  Relational Operator1/1 -> Sum/2
  Relational Operator/1 -> Sum/1
  Sum/1 -> out_1/1

== system OMSv1_4/OMS v1.4  12/31/07/IM CN-LMLN/Saccade Enable/Ret FB sample/event timer2/SampHold?1/Sign ==
  in_1 : Inport  OutDataType=sfix(16)  OutScaling=2^0
  Constant : Constant  Value=0  OutDataType=sfix(16)  OutScaling=2^0
  Relational Operator : RelationalOperator  Operator=>  InputSameDT=on
  Relational Operator1 : RelationalOperator  Operator=<  InputSameDT=on
  Sum : Sum  Inputs=+-  OutDataType=sfix(16)  OutScaling=2^0  SaturateOnIntegerOverflow=on  InputSameDT=on
  out_1 : Outport  OutDataType=sfix(16)  OutScaling=2^0  InitialOutput=0
  wires:
  in_1/1 -> Relational Operator/1, Relational Operator1/1
  Constant/1 -> Relational Operator1/2, Relational Operator/2
  Relational Operator1/1 -> Sum/2
  Relational Operator/1 -> Sum/1
  Sum/1 -> out_1/1

== system OMSv1_4/OMS v1.4  12/31/07/IM CN-LMLN/Saccade Enable/Ret FB sample/event timer2/leading edge detect/Sign ==
  in_1 : Inport  OutDataType=sfix(16)  OutScaling=2^0
  Constant : Constant  Value=0  OutDataType=sfix(16)  OutScaling=2^0
  Relational Operator : RelationalOperator  Operator=>  InputSameDT=on
  Relational Operator1 : RelationalOperator  Operator=<  InputSameDT=on
  Sum : Sum  Inputs=+-  OutDataType=sfix(16)  OutScaling=2^0  SaturateOnIntegerOverflow=on  InputSameDT=on
  out_1 : Outport  OutDataType=sfix(16)  OutScaling=2^0  InitialOutput=0
  wires:
  in_1/1 -> Relational Operator/1, Relational Operator1/1
  Constant/1 -> Relational Operator1/2, Relational Operator/2
  Relational Operator1/1 -> Sum/2
  Relational Operator/1 -> Sum/1
  Sum/1 -> out_1/1

== system OMSv1_4/OMS v1.4  12/31/07/IM CN-LMLN/Saccade Enable/Ret FB sample/event timer2/trailing edge detect/Sign ==
  in_1 : Inport  OutDataType=sfix(16)  OutScaling=2^0
  Constant : Constant  Value=0  OutDataType=sfix(16)  OutScaling=2^0
  Relational Operator : RelationalOperator  Operator=>  InputSameDT=on
  Relational Operator1 : RelationalOperator  Operator=<  InputSameDT=on
  Sum : Sum  Inputs=+-  OutDataType=sfix(16)  OutScaling=2^0  SaturateOnIntegerOverflow=on  InputSameDT=on
  out_1 : Outport  OutDataType=sfix(16)  OutScaling=2^0  InitialOutput=0
  wires:
  Sum/1 -> out_1/1
  Relational Operator/1 -> Sum/1
  Relational Operator1/1 -> Sum/2
  Constant/1 -> Relational Operator1/2, Relational Operator/2
  in_1/1 -> Relational Operator/1, Relational Operator1/1

== system OMSv1_4/OMS v1.4  12/31/07/IM CN-LMLN/Saccade Enable/Ret FB sample/event timer3/SampHold?1/Sign ==
  in_1 : Inport  OutDataType=sfix(16)  OutScaling=2^0
  Constant : Constant  Value=0  OutDataType=sfix(16)  OutScaling=2^0
  Relational Operator : RelationalOperator  Operator=>  InputSameDT=on
  Relational Operator1 : RelationalOperator  Operator=<  InputSameDT=on
  Sum : Sum  Inputs=+-  OutDataType=sfix(16)  OutScaling=2^0  SaturateOnIntegerOverflow=on  InputSameDT=on
  out_1 : Outport  OutDataType=sfix(16)  OutScaling=2^0  InitialOutput=0
  wires:
  Sum/1 -> out_1/1
  Relational Operator/1 -> Sum/1
  Relational Operator1/1 -> Sum/2
  Constant/1 -> Relational Operator1/2, Relational Operator/2
  in_1/1 -> Relational Operator/1, Relational Operator1/1

== system OMSv1_4/OMS v1.4  12/31/07/IM CN-LMLN/Saccade Enable/Ret FB sample/event timer3/leading edge detect/Sign ==
  in_1 : Inport  OutDataType=sfix(16)  OutScaling=2^0
  Constant : Constant  Value=0  OutDataType=sfix(16)  OutScaling=2^0
  Relational Operator : RelationalOperator  Operator=>  InputSameDT=on
  Relational Operator1 : RelationalOperator  Operator=<  InputSameDT=on
  Sum : Sum  Inputs=+-  OutDataType=sfix(16)  OutScaling=2^0  SaturateOnIntegerOverflow=on  InputSameDT=on
  out_1 : Outport  OutDataType=sfix(16)  OutScaling=2^0  InitialOutput=0
  wires:
  Sum/1 -> out_1/1
  Relational Operator/1 -> Sum/1
  Relational Operator1/1 -> Sum/2
  Constant/1 -> Relational Operator1/2, Relational Operator/2
  in_1/1 -> Relational Operator/1, Relational Operator1/1

== system OMSv1_4/OMS v1.4  12/31/07/IM CN-LMLN/Saccade Enable/Ret FB sample/event timer3/trailing edge detect/Sign ==
  in_1 : Inport  OutDataType=sfix(16)  OutScaling=2^0
  Constant : Constant  Value=0  OutDataType=sfix(16)  OutScaling=2^0
  Relational Operator : RelationalOperator  Operator=>  InputSameDT=on
  Relational Operator1 : RelationalOperator  Operator=<  InputSameDT=on
  Sum : Sum  Inputs=+-  OutDataType=sfix(16)  OutScaling=2^0  SaturateOnIntegerOverflow=on  InputSameDT=on
  out_1 : Outport  OutDataType=sfix(16)  OutScaling=2^0  InitialOutput=0
  wires:
  in_1/1 -> Relational Operator/1, Relational Operator1/1
  Constant/1 -> Relational Operator1/2, Relational Operator/2
  Relational Operator1/1 -> Sum/2
  Relational Operator/1 -> Sum/1
  Sum/1 -> out_1/1

== system OMSv1_4/OMS v1.4  12/31/07/IM CN-LMLN/Saccade Motor Commmand/TCHNG Override/event timer2/SampHold?1/Sign ==
  in_1 : Inport  OutDataType=sfix(16)  OutScaling=2^0
  Constant : Constant  Value=0  OutDataType=sfix(16)  OutScaling=2^0
  Relational Operator : RelationalOperator  Operator=>  InputSameDT=on
  Relational Operator1 : RelationalOperator  Operator=<  InputSameDT=on
  Sum : Sum  Inputs=+-  OutDataType=sfix(16)  OutScaling=2^0  SaturateOnIntegerOverflow=on  InputSameDT=on
  out_1 : Outport  OutDataType=sfix(16)  OutScaling=2^0  InitialOutput=0
  wires:
  in_1/1 -> Relational Operator1/1, Relational Operator/1
  Constant/1 -> Relational Operator/2, Relational Operator1/2
  Relational Operator1/1 -> Sum/2
  Relational Operator/1 -> Sum/1
  Sum/1 -> out_1/1

== system OMSv1_4/OMS v1.4  12/31/07/IM CN-LMLN/Saccade Motor Commmand/TCHNG Override/event timer2/leading edge detect/Sign ==
  in_1 : Inport  OutDataType=sfix(16)  OutScaling=2^0
  Constant : Constant  Value=0  OutDataType=sfix(16)  OutScaling=2^0
  Relational Operator : RelationalOperator  Operator=>  InputSameDT=on
  Relational Operator1 : RelationalOperator  Operator=<  InputSameDT=on
  Sum : Sum  Inputs=+-  OutDataType=sfix(16)  OutScaling=2^0  SaturateOnIntegerOverflow=on  InputSameDT=on
  out_1 : Outport  OutDataType=sfix(16)  OutScaling=2^0  InitialOutput=0
  wires:
  in_1/1 -> Relational Operator1/1, Relational Operator/1
  Constant/1 -> Relational Operator/2, Relational Operator1/2
  Relational Operator1/1 -> Sum/2
  Relational Operator/1 -> Sum/1
  Sum/1 -> out_1/1

== system OMSv1_4/OMS v1.4  12/31/07/IM CN-LMLN/Saccade Motor Commmand/TCHNG Override/event timer2/trailing edge detect/Sign ==
  in_1 : Inport  OutDataType=sfix(16)  OutScaling=2^0
  Constant : Constant  Value=0  OutDataType=sfix(16)  OutScaling=2^0
  Relational Operator : RelationalOperator  Operator=>  InputSameDT=on
  Relational Operator1 : RelationalOperator  Operator=<  InputSameDT=on
  Sum : Sum  Inputs=+-  OutDataType=sfix(16)  OutScaling=2^0  SaturateOnIntegerOverflow=on  InputSameDT=on
  out_1 : Outport  OutDataType=sfix(16)  OutScaling=2^0  InitialOutput=0
  wires:
  Sum/1 -> out_1/1
  Relational Operator/1 -> Sum/1
  Relational Operator1/1 -> Sum/2
  Constant/1 -> Relational Operator/2, Relational Operator1/2
  in_1/1 -> Relational Operator1/1, Relational Operator/1

== system OMSv1_4/OMS v1.4  12/31/07/IM CN-LMLN/Saccade Motor Commmand/Voluntary Saccade Switch1/TCHNG Override2/event timer2/Latch1 ==
  in_1 : Inport  OutDataType=sfix(16)  OutScaling=2^0
  in_2 : Inport  Port=2  OutDataType=sfix(16)  OutScaling=2^0
  Demux : Demux  Outputs=2
  Logic : CombinatorialLogic  TruthTable=[0 1;0 1;1 0;0 1;1 0;0 1;1 0;1 0]
  Memory : Memory  Orientation=left  X0=ini
  Mux : Mux  Inputs=3
  out_1 : Outport  OutDataType=sfix(16)  OutScaling=2^0  InitialOutput=0
  out_2 : Outport  Port=2  OutDataType=sfix(16)  OutScaling=2^0  InitialOutput=0
  wires:
  in_2/1 -> Mux/3
  in_1/1 -> Mux/2
  Memory/1 -> Mux/1
  Demux/1 -> Memory/1, out_1/1
  Mux/1 -> Logic/1
  Logic/1 -> Demux/1
  Demux/2 -> out_2/1

== system OMSv1_4/OMS v1.4  12/31/07/IM CN-LMLN/Saccade Motor Commmand/Voluntary Saccade Switch1/TCHNG Override2/event timer2/SampHold?1 ==
  note: When "S/H?" is LOW, then "Input" is switched directly to the
      | output ("sample").  When "S/H?" is HIGH, the current output is
      | maintained ("hold").
  Input : Inport  OutDataType=sfix(16)  OutScaling=2^0
  S/H? : Inport  Port=2  OutDataType=sfix(16)  OutScaling=2^0
  Memory : Memory  Orientation=left
  Sign : Subsystem
      mask Type: Sign
      mask Description: y = sign(x)
      mask Help: Sign Function:\n\t\t\ty = 1 if x > 0\n\t\t\ty = 0 if x = 0\n\t\t\ty = -1 if x < 0
      mask Display: plot(-50,-50,50,50,[-50,50],[0,0],[0,0],[-50,50],[-40,0],[-30,-30],[0,40],[30,30])
  Switch2 : Switch  Threshold=0.5  SaturateOnIntegerOverflow=on  InputSameDT=on
  output : Outport  OutDataType=sfix(16)  OutScaling=2^0  InitialOutput=0
  wires:
  Switch2/1 -> Memory/1, output/1
  Sign/1(out_1) -> Switch2/2
  S/H?/1 -> Sign/1(in_1)
  Memory/1 -> Switch2/1
  Input/1 -> Switch2/3

== system OMSv1_4/OMS v1.4  12/31/07/IM CN-LMLN/Saccade Motor Commmand/Voluntary Saccade Switch1/TCHNG Override2/event timer2/leading edge detect ==
  note: It is also possible to remove the SIGNUM function
      | and the '==', and replace them with a simple
      | switch with a threshold of (say) 150 or so.
  note: leading edge detection
  in_1 : Inport  OutDataType=sfix(16)  OutScaling=2^0
  Abs : Abs  SaturateOnIntegerOverflow=on
  Derivative : Derivative
  Relational Operator : RelationalOperator  Operator===  InputSameDT=on
  Sign : Subsystem
      mask Type: Sign
      mask Description: y = sign(x)
      mask Help: Sign Function:\n\t\t\ty = 1 if x > 0\n\t\t\ty = 0 if x = 0\n\t\t\ty = -1 if x < 0
      mask Display: plot(-50,-50,50,50,[-50,50],[0,0],[0,0],[-50,50],[-40,0],[-30,-30],[0,40],[30,30])
  Threshold 1 : Constant  OutDataType=sfix(16)  OutScaling=2^0
  out_1 : Outport  OutDataType=sfix(16)  OutScaling=2^0  InitialOutput=0
  wires:
  Abs/1 -> Derivative/1
  Derivative/1 -> Sign/1(in_1)
  Sign/1(out_1) -> Relational Operator/1
  Threshold 1/1 -> Relational Operator/2
  Relational Operator/1 -> out_1/1
  in_1/1 -> Abs/1

== system OMSv1_4/OMS v1.4  12/31/07/IM CN-LMLN/Saccade Motor Commmand/Voluntary Saccade Switch1/TCHNG Override2/event timer2/trailing edge detect ==
  note: trailing edge detection
  note: It is also possible to remove the SIGNUM function
      | and the '==', and replace them with a simple
      | switch with a threshold of (say) 150 or so.
  in_1 : Inport  OutDataType=sfix(16)  OutScaling=2^0
  Abs : Abs  SaturateOnIntegerOverflow=on
  Derivative : Derivative
  Relational Operator : RelationalOperator  Operator===  InputSameDT=on
  Sign : Subsystem
      mask Type: Sign
      mask Description: y = sign(x)
      mask Help: Sign Function:\n\t\t\ty = 1 if x > 0\n\t\t\ty = 0 if x = 0\n\t\t\ty = -1 if x < 0
      mask Display: plot(-50,-50,50,50,[-50,50],[0,0],[0,0],[-50,50],[-40,0],[-30,-30],[0,40],[30,30])
  Threshold 1 : Constant  Value=-1  OutDataType=sfix(16)  OutScaling=2^0
  out_1 : Outport  OutDataType=sfix(16)  OutScaling=2^0  InitialOutput=0
  wires:
  in_1/1 -> Abs/1
  Relational Operator/1 -> out_1/1
  Threshold 1/1 -> Relational Operator/2
  Sign/1(out_1) -> Relational Operator/1
  Derivative/1 -> Sign/1(in_1)
  Abs/1 -> Derivative/1

== system OMSv1_4/OMS v1.4  12/31/07/IM CN-LMLN/Saccade Motor Commmand/Voluntary Saccade Switch1/TCHNG Override2/leading edge detect/Sign ==
  in_1 : Inport  OutDataType=sfix(16)  OutScaling=2^0
  Constant : Constant  Value=0  OutDataType=sfix(16)  OutScaling=2^0
  Relational Operator : RelationalOperator  Operator=>  InputSameDT=on
  Relational Operator1 : RelationalOperator  Operator=<  InputSameDT=on
  Sum : Sum  Inputs=+-  OutDataType=sfix(16)  OutScaling=2^0  SaturateOnIntegerOverflow=on  InputSameDT=on
  out_1 : Outport  OutDataType=sfix(16)  OutScaling=2^0  InitialOutput=0
  wires:
  Sum/1 -> out_1/1
  Relational Operator/1 -> Sum/1
  Relational Operator1/1 -> Sum/2
  Constant/1 -> Relational Operator/2, Relational Operator1/2
  in_1/1 -> Relational Operator1/1, Relational Operator/1

== system OMSv1_4/OMS v1.4  12/31/07/IM CN-LMLN/Saccade Motor Commmand/Voluntary Saccade Switch1/prolong2/SampHold?2/Sign ==
  in_1 : Inport  OutDataType=sfix(16)  OutScaling=2^0
  Constant : Constant  Value=0  OutDataType=sfix(16)  OutScaling=2^0
  Relational Operator : RelationalOperator  Operator=>  InputSameDT=on
  Relational Operator1 : RelationalOperator  Operator=<  InputSameDT=on
  Sum : Sum  Inputs=+-  OutDataType=sfix(16)  OutScaling=2^0  SaturateOnIntegerOverflow=on  InputSameDT=on
  out_1 : Outport  OutDataType=sfix(16)  OutScaling=2^0  InitialOutput=0
  wires:
  in_1/1 -> Relational Operator/1, Relational Operator1/1
  Constant/1 -> Relational Operator1/2, Relational Operator/2
  Relational Operator1/1 -> Sum/2
  Relational Operator/1 -> Sum/1
  Sum/1 -> out_1/1

== system OMSv1_4/OMS v1.4  12/31/07/IM CN-LMLN/Saccade Motor Commmand/Voluntary Saccade Switch1/prolong2/leading edge detect/Sign ==
  in_1 : Inport  OutDataType=sfix(16)  OutScaling=2^0
  Constant : Constant  Value=0  OutDataType=sfix(16)  OutScaling=2^0
  Relational Operator : RelationalOperator  Operator=>  InputSameDT=on
  Relational Operator1 : RelationalOperator  Operator=<  InputSameDT=on
  Sum : Sum  Inputs=+-  OutDataType=sfix(16)  OutScaling=2^0  SaturateOnIntegerOverflow=on  InputSameDT=on
  out_1 : Outport  OutDataType=sfix(16)  OutScaling=2^0  InitialOutput=0
  wires:
  Sum/1 -> out_1/1
  Relational Operator/1 -> Sum/1
  Relational Operator1/1 -> Sum/2
  Constant/1 -> Relational Operator/2, Relational Operator1/2
  in_1/1 -> Relational Operator1/1, Relational Operator/1

== system OMSv1_4/OMS v1.4  12/31/07/IM CN-LMLN/Saccade Motor Commmand/Voluntary Saccade Switch1/prolong2/trailing edge detect/Sign ==
  in_1 : Inport  OutDataType=sfix(16)  OutScaling=2^0
  Constant : Constant  Value=0  OutDataType=sfix(16)  OutScaling=2^0
  Relational Operator : RelationalOperator  Operator=>  InputSameDT=on
  Relational Operator1 : RelationalOperator  Operator=<  InputSameDT=on
  Sum : Sum  Inputs=+-  OutDataType=sfix(16)  OutScaling=2^0  SaturateOnIntegerOverflow=on  InputSameDT=on
  out_1 : Outport  OutDataType=sfix(16)  OutScaling=2^0  InitialOutput=0
  wires:
  in_1/1 -> Relational Operator/1, Relational Operator1/1
  Constant/1 -> Relational Operator1/2, Relational Operator/2
  Relational Operator1/1 -> Sum/2
  Relational Operator/1 -> Sum/1
  Sum/1 -> out_1/1

== system OMSv1_4/OMS v1.4  12/31/07/IM CN-LMLN/BS/FS Logic/BS Enable1/BS Timing/event timer2/SampHold?1/Sign ==
  in_1 : Inport  OutDataType=sfix(16)  OutScaling=2^0
  Constant : Constant  Value=0  OutDataType=sfix(16)  OutScaling=2^0
  Relational Operator : RelationalOperator  Operator=>  InputSameDT=on
  Relational Operator1 : RelationalOperator  Operator=<  InputSameDT=on
  Sum : Sum  Inputs=+-  OutDataType=sfix(16)  OutScaling=2^0  SaturateOnIntegerOverflow=on  InputSameDT=on
  out_1 : Outport  OutDataType=sfix(16)  OutScaling=2^0  InitialOutput=0
  wires:
  in_1/1 -> Relational Operator1/1, Relational Operator/1
  Constant/1 -> Relational Operator/2, Relational Operator1/2
  Relational Operator1/1 -> Sum/2
  Relational Operator/1 -> Sum/1
  Sum/1 -> out_1/1

== system OMSv1_4/OMS v1.4  12/31/07/IM CN-LMLN/BS/FS Logic/BS Enable1/BS Timing/event timer2/leading edge detect/Sign ==
  in_1 : Inport  OutDataType=sfix(16)  OutScaling=2^0
  Constant : Constant  Value=0  OutDataType=sfix(16)  OutScaling=2^0
  Relational Operator : RelationalOperator  Operator=>  InputSameDT=on
  Relational Operator1 : RelationalOperator  Operator=<  InputSameDT=on
  Sum : Sum  Inputs=+-  OutDataType=sfix(16)  OutScaling=2^0  SaturateOnIntegerOverflow=on  InputSameDT=on
  out_1 : Outport  OutDataType=sfix(16)  OutScaling=2^0  InitialOutput=0
  wires:
  in_1/1 -> Relational Operator1/1, Relational Operator/1
  Constant/1 -> Relational Operator/2, Relational Operator1/2
  Relational Operator1/1 -> Sum/2
  Relational Operator/1 -> Sum/1
  Sum/1 -> out_1/1
